simulink model "MultipleAgentsChoice_NoVR"  (R2013b)
settings: Solver=ode45  StartTime=0.0  StopTime=1000  RelTol=1e-4  AbsTol=1e-4
libraries: simulink x24
(part 5 of 5)

== system MultipleAgentsChoice_NoVR/StatePropagation/SatelliteControlAccel/Agent Body3/Actual Thruster response/Ythruster1/Thruster1/ThrustBlock ==
  ForceRequest : Inport
  Short? : Inport  Port=2
  MainSwitch : Inport  Port=3
  Feed : Inport  Port=4
  CathodeEfficiency : Inport  Port=5
  ActiveThruster (logical) : Subsystem
  Bus Creator : BusCreator  Inputs=2
  Product : Product  RndMeth=Zero
  Product1 : Product  RndMeth=Zero
  Voltage/Current : Subsystem
  OutputForce : Outport
  ThrusterData : Outport  Port=2
  wires:
  [CathodeEfficiency] -> Product1/2
  Product/1 -> Product1/1
  [ForceRequest] -> Product/2
  CathodeEfficiency/1 -> [CathodeEfficiency]
  ForceRequest/1 -> [ForceRequest]
  ActiveThruster (logical)/1(Active) -> Product/1
  Bus Creator/1 -> ThrusterData/1
  Voltage/Current/2(Current) -> Bus Creator/2  "current"
  Voltage/Current/1(Voltage) -> Bus Creator/1  "voltage"
  Feed/1 -> ActiveThruster (logical)/3(Feed?), Voltage/Current/3(Feed?)
  Short?/1 -> Voltage/Current/1(Short?), ActiveThruster (logical)/1(Short?)
  MainSwitch/1 -> Voltage/Current/2(MainSwitch), ActiveThruster (logical)/2(ThrusterOn?)
  Product1/1 -> OutputForce/1

== system MultipleAgentsChoice_NoVR/StatePropagation/SatelliteControlAccel/Agent Body3/Actual Thruster response/Zthruster1/Thruster1/ForceShort ==
  note: Detect event and introduce short, otherwise pass through current result of short status
  Event : Inport
  SC : Inport  Port=2
  MainSwitch : Inport  Port=3
  Constant : Constant
  Data Type Conversion : DataTypeConversion
  Detect Increase : simulink/Logic and Bit Operations/Detect Increase  vinit=0  InputProcessing=Inherited  OutDataTypeStr=uint8
  Multiport Switch : MultiPortSwitch  DataPortOrder=Zero-based contiguous  Inputs=2  zeroidx=on
  S/C Conditioning : Subsystem
  SC_out : Outport
  wires:
  Event/1 -> Detect Increase/1
  Detect Increase/1 -> Data Type Conversion/1
  S/C Conditioning/1(Short?) -> SC_out/1
  MainSwitch/1 -> S/C Conditioning/2(MainSwitch)
  Data Type Conversion/1 -> Multiport Switch/1
  SC/1 -> Multiport Switch/2
  Constant/1 -> Multiport Switch/3
  Multiport Switch/1 -> S/C Conditioning/1(SC)

== system MultipleAgentsChoice_NoVR/StatePropagation/SatelliteControlAccel/Agent Body3/Actual Thruster response/Zthruster1/Thruster1/ThrustBlock ==
  ForceRequest : Inport
  Short? : Inport  Port=2
  MainSwitch : Inport  Port=3
  Feed : Inport  Port=4
  CathodeEfficiency : Inport  Port=5
  ActiveThruster (logical) : Subsystem
  Bus Creator : BusCreator  Inputs=2
  Product : Product  RndMeth=Zero
  Product1 : Product  RndMeth=Zero
  Voltage/Current : Subsystem
  OutputForce : Outport
  ThrusterData : Outport  Port=2
  wires:
  MainSwitch/1 -> ActiveThruster (logical)/2(ThrusterOn?), Voltage/Current/2(MainSwitch)
  Short?/1 -> ActiveThruster (logical)/1(Short?), Voltage/Current/1(Short?)
  Feed/1 -> Voltage/Current/3(Feed?), ActiveThruster (logical)/3(Feed?)
  Voltage/Current/1(Voltage) -> Bus Creator/1  "voltage"
  Voltage/Current/2(Current) -> Bus Creator/2  "current"
  Bus Creator/1 -> ThrusterData/1
  ActiveThruster (logical)/1(Active) -> Product/1
  ForceRequest/1 -> [ForceRequest]
  CathodeEfficiency/1 -> [CathodeEfficiency]
  [ForceRequest] -> Product/2
  Product/1 -> Product1/1
  [CathodeEfficiency] -> Product1/2
  Product1/1 -> OutputForce/1

== system MultipleAgentsChoice_NoVR/StatePropagation/SatelliteControlAccel/Agent Body1/Actual Thruster response/XYZthruster/Thruster1/ForceShort/S//C Conditioning ==
  SC : Inport
  MainSwitch : Inport  Port=2
  Constant : Constant  Value=2
  Data Type Conversion : DataTypeConversion
  Detect Decrease : simulink/Logic and Bit Operations/Detect Decrease  vinit=0  InputProcessing=Inherited  OutDataTypeStr=uint8
  Multiport Switch : MultiPortSwitch  DataPortOrder=Zero-based contiguous  Inputs=2  zeroidx=on
  Short? : Outport
  wires:
  MainSwitch/1 -> Detect Decrease/1
  Detect Decrease/1 -> Data Type Conversion/1
  Data Type Conversion/1 -> Multiport Switch/1
  SC/1 -> Multiport Switch/2
  Constant/1 -> Multiport Switch/3
  Multiport Switch/1 -> Short?/1

== system MultipleAgentsChoice_NoVR/StatePropagation/SatelliteControlAccel/Agent Body1/Actual Thruster response/XYZthruster/Thruster1/ThrustBlock/ActiveThruster (logical) ==
  Short? : Inport
  ThrusterOn? : Inport  Port=2
  Feed? : Inport  Port=3
  MATLAB Fcn : MATLABFcn  MATLABFcn=ActiveThruster  OutputDimensions=1
  Mux : Mux  Inputs=3
  Active : Outport
  wires:
  Short?/1 -> Mux/1
  ThrusterOn?/1 -> Mux/2
  Feed?/1 -> Mux/3
  Mux/1 -> MATLAB Fcn/1
  MATLAB Fcn/1 -> Active/1

== system MultipleAgentsChoice_NoVR/StatePropagation/SatelliteControlAccel/Agent Body1/Actual Thruster response/XYZthruster/Thruster1/ThrustBlock/Voltage//Current ==
  Short? : Inport
  MainSwitch : Inport  Port=2
  Feed? : Inport  Port=3
  Demux : Demux  Outputs=2
  MATLAB Fcn : MATLABFcn  MATLABFcn=ThrusterData  OutputDimensions=2
  Mux : Mux  Inputs=3
  Voltage : Outport
  Current : Outport  Port=2
  wires:
  Short?/1 -> Mux/1
  MainSwitch/1 -> Mux/2
  Feed?/1 -> Mux/3
  Mux/1 -> MATLAB Fcn/1
  MATLAB Fcn/1 -> Demux/1
  Demux/1 -> Voltage/1
  Demux/2 -> Current/1

== system MultipleAgentsChoice_NoVR/StatePropagation/SatelliteControlAccel/Agent Body1/Actual Thruster response/Xthruster/Thruster1/ForceShort/S//C Conditioning ==
  SC : Inport
  MainSwitch : Inport  Port=2
  Constant : Constant  Value=2
  Data Type Conversion : DataTypeConversion
  Detect Decrease : simulink/Logic and Bit Operations/Detect Decrease  vinit=0  InputProcessing=Inherited  OutDataTypeStr=uint8
  Multiport Switch : MultiPortSwitch  DataPortOrder=Zero-based contiguous  Inputs=2  zeroidx=on
  Short? : Outport
  wires:
  Multiport Switch/1 -> Short?/1
  Constant/1 -> Multiport Switch/3
  SC/1 -> Multiport Switch/2
  Data Type Conversion/1 -> Multiport Switch/1
  Detect Decrease/1 -> Data Type Conversion/1
  MainSwitch/1 -> Detect Decrease/1

== system MultipleAgentsChoice_NoVR/StatePropagation/SatelliteControlAccel/Agent Body1/Actual Thruster response/Xthruster/Thruster1/ThrustBlock/ActiveThruster (logical) ==
  Short? : Inport
  ThrusterOn? : Inport  Port=2
  Feed? : Inport  Port=3
  MATLAB Fcn : MATLABFcn  MATLABFcn=ActiveThruster  OutputDimensions=1
  Mux : Mux  Inputs=3
  Active : Outport
  wires:
  MATLAB Fcn/1 -> Active/1
  Mux/1 -> MATLAB Fcn/1
  Feed?/1 -> Mux/3
  ThrusterOn?/1 -> Mux/2
  Short?/1 -> Mux/1

== system MultipleAgentsChoice_NoVR/StatePropagation/SatelliteControlAccel/Agent Body1/Actual Thruster response/Xthruster/Thruster1/ThrustBlock/Voltage//Current ==
  Short? : Inport
  MainSwitch : Inport  Port=2
  Feed? : Inport  Port=3
  Demux : Demux  Outputs=2
  MATLAB Fcn : MATLABFcn  MATLABFcn=ThrusterData  OutputDimensions=2
  Mux : Mux  Inputs=3
  Voltage : Outport
  Current : Outport  Port=2
  wires:
  Demux/2 -> Current/1
  Demux/1 -> Voltage/1
  MATLAB Fcn/1 -> Demux/1
  Mux/1 -> MATLAB Fcn/1
  Feed?/1 -> Mux/3
  MainSwitch/1 -> Mux/2
  Short?/1 -> Mux/1

== system MultipleAgentsChoice_NoVR/StatePropagation/SatelliteControlAccel/Agent Body1/Actual Thruster response/Ythruster1/Thruster1/ForceShort/S//C Conditioning ==
  SC : Inport
  MainSwitch : Inport  Port=2
  Constant : Constant  Value=2
  Data Type Conversion : DataTypeConversion
  Detect Decrease : simulink/Logic and Bit Operations/Detect Decrease  vinit=0  InputProcessing=Inherited  OutDataTypeStr=uint8
  Multiport Switch : MultiPortSwitch  DataPortOrder=Zero-based contiguous  Inputs=2  zeroidx=on
  Short? : Outport
  wires:
  MainSwitch/1 -> Detect Decrease/1
  Detect Decrease/1 -> Data Type Conversion/1
  Data Type Conversion/1 -> Multiport Switch/1
  SC/1 -> Multiport Switch/2
  Constant/1 -> Multiport Switch/3
  Multiport Switch/1 -> Short?/1

== system MultipleAgentsChoice_NoVR/StatePropagation/SatelliteControlAccel/Agent Body1/Actual Thruster response/Ythruster1/Thruster1/ThrustBlock/ActiveThruster (logical) ==
  Short? : Inport
  ThrusterOn? : Inport  Port=2
  Feed? : Inport  Port=3
  MATLAB Fcn : MATLABFcn  MATLABFcn=ActiveThruster  OutputDimensions=1
  Mux : Mux  Inputs=3
  Active : Outport
  wires:
  Short?/1 -> Mux/1
  ThrusterOn?/1 -> Mux/2
  Feed?/1 -> Mux/3
  Mux/1 -> MATLAB Fcn/1
  MATLAB Fcn/1 -> Active/1

== system MultipleAgentsChoice_NoVR/StatePropagation/SatelliteControlAccel/Agent Body1/Actual Thruster response/Ythruster1/Thruster1/ThrustBlock/Voltage//Current ==
  Short? : Inport
  MainSwitch : Inport  Port=2
  Feed? : Inport  Port=3
  Demux : Demux  Outputs=2
  MATLAB Fcn : MATLABFcn  MATLABFcn=ThrusterData  OutputDimensions=2
  Mux : Mux  Inputs=3
  Voltage : Outport
  Current : Outport  Port=2
  wires:
  Short?/1 -> Mux/1
  MainSwitch/1 -> Mux/2
  Feed?/1 -> Mux/3
  Mux/1 -> MATLAB Fcn/1
  MATLAB Fcn/1 -> Demux/1
  Demux/1 -> Voltage/1
  Demux/2 -> Current/1

== system MultipleAgentsChoice_NoVR/StatePropagation/SatelliteControlAccel/Agent Body1/Actual Thruster response/Zthruster1/Thruster1/ForceShort/S//C Conditioning ==
  SC : Inport
  MainSwitch : Inport  Port=2
  Constant : Constant  Value=2
  Data Type Conversion : DataTypeConversion
  Detect Decrease : simulink/Logic and Bit Operations/Detect Decrease  vinit=0  InputProcessing=Inherited  OutDataTypeStr=uint8
  Multiport Switch : MultiPortSwitch  DataPortOrder=Zero-based contiguous  Inputs=2  zeroidx=on
  Short? : Outport
  wires:
  Multiport Switch/1 -> Short?/1
  Constant/1 -> Multiport Switch/3
  SC/1 -> Multiport Switch/2
  Data Type Conversion/1 -> Multiport Switch/1
  Detect Decrease/1 -> Data Type Conversion/1
  MainSwitch/1 -> Detect Decrease/1

== system MultipleAgentsChoice_NoVR/StatePropagation/SatelliteControlAccel/Agent Body1/Actual Thruster response/Zthruster1/Thruster1/ThrustBlock/ActiveThruster (logical) ==
  Short? : Inport
  ThrusterOn? : Inport  Port=2
  Feed? : Inport  Port=3
  MATLAB Fcn : MATLABFcn  MATLABFcn=ActiveThruster  OutputDimensions=1
  Mux : Mux  Inputs=3
  Active : Outport
  wires:
  MATLAB Fcn/1 -> Active/1
  Mux/1 -> MATLAB Fcn/1
  Feed?/1 -> Mux/3
  ThrusterOn?/1 -> Mux/2
  Short?/1 -> Mux/1

== system MultipleAgentsChoice_NoVR/StatePropagation/SatelliteControlAccel/Agent Body1/Actual Thruster response/Zthruster1/Thruster1/ThrustBlock/Voltage//Current ==
  Short? : Inport
  MainSwitch : Inport  Port=2
  Feed? : Inport  Port=3
  Demux : Demux  Outputs=2
  MATLAB Fcn : MATLABFcn  MATLABFcn=ThrusterData  OutputDimensions=2
  Mux : Mux  Inputs=3
  Voltage : Outport
  Current : Outport  Port=2
  wires:
  Demux/2 -> Current/1
  Demux/1 -> Voltage/1
  MATLAB Fcn/1 -> Demux/1
  Mux/1 -> MATLAB Fcn/1
  Feed?/1 -> Mux/3
  MainSwitch/1 -> Mux/2
  Short?/1 -> Mux/1

== system MultipleAgentsChoice_NoVR/StatePropagation/SatelliteControlAccel/Agent Body2/Actual Thruster response/XYZthruster/Thruster1/ForceShort/S//C Conditioning ==
  SC : Inport
  MainSwitch : Inport  Port=2
  Constant : Constant  Value=2
  Data Type Conversion : DataTypeConversion
  Detect Decrease : simulink/Logic and Bit Operations/Detect Decrease  vinit=0  InputProcessing=Inherited  OutDataTypeStr=uint8
  Multiport Switch : MultiPortSwitch  DataPortOrder=Zero-based contiguous  Inputs=2  zeroidx=on
  Short? : Outport
  wires:
  Multiport Switch/1 -> Short?/1
  Constant/1 -> Multiport Switch/3
  SC/1 -> Multiport Switch/2
  Data Type Conversion/1 -> Multiport Switch/1
  Detect Decrease/1 -> Data Type Conversion/1
  MainSwitch/1 -> Detect Decrease/1

== system MultipleAgentsChoice_NoVR/StatePropagation/SatelliteControlAccel/Agent Body2/Actual Thruster response/XYZthruster/Thruster1/ThrustBlock/ActiveThruster (logical) ==
  Short? : Inport
  ThrusterOn? : Inport  Port=2
  Feed? : Inport  Port=3
  MATLAB Fcn : MATLABFcn  MATLABFcn=ActiveThruster  OutputDimensions=1
  Mux : Mux  Inputs=3
  Active : Outport
  wires:
  MATLAB Fcn/1 -> Active/1
  Mux/1 -> MATLAB Fcn/1
  Feed?/1 -> Mux/3
  ThrusterOn?/1 -> Mux/2
  Short?/1 -> Mux/1

== system MultipleAgentsChoice_NoVR/StatePropagation/SatelliteControlAccel/Agent Body2/Actual Thruster response/XYZthruster/Thruster1/ThrustBlock/Voltage//Current ==
  Short? : Inport
  MainSwitch : Inport  Port=2
  Feed? : Inport  Port=3
  Demux : Demux  Outputs=2
  MATLAB Fcn : MATLABFcn  MATLABFcn=ThrusterData  OutputDimensions=2
  Mux : Mux  Inputs=3
  Voltage : Outport
  Current : Outport  Port=2
  wires:
  Demux/2 -> Current/1
  Demux/1 -> Voltage/1
  MATLAB Fcn/1 -> Demux/1
  Mux/1 -> MATLAB Fcn/1
  Feed?/1 -> Mux/3
  MainSwitch/1 -> Mux/2
  Short?/1 -> Mux/1

== system MultipleAgentsChoice_NoVR/StatePropagation/SatelliteControlAccel/Agent Body2/Actual Thruster response/Xthruster/Thruster1/ForceShort/S//C Conditioning ==
  SC : Inport
  MainSwitch : Inport  Port=2
  Constant : Constant  Value=2
  Data Type Conversion : DataTypeConversion
  Detect Decrease : simulink/Logic and Bit Operations/Detect Decrease  vinit=0  InputProcessing=Inherited  OutDataTypeStr=uint8
  Multiport Switch : MultiPortSwitch  DataPortOrder=Zero-based contiguous  Inputs=2  zeroidx=on
  Short? : Outport
  wires:
  MainSwitch/1 -> Detect Decrease/1
  Detect Decrease/1 -> Data Type Conversion/1
  Data Type Conversion/1 -> Multiport Switch/1
  SC/1 -> Multiport Switch/2
  Constant/1 -> Multiport Switch/3
  Multiport Switch/1 -> Short?/1

== system MultipleAgentsChoice_NoVR/StatePropagation/SatelliteControlAccel/Agent Body2/Actual Thruster response/Xthruster/Thruster1/ThrustBlock/ActiveThruster (logical) ==
  Short? : Inport
  ThrusterOn? : Inport  Port=2
  Feed? : Inport  Port=3
  MATLAB Fcn : MATLABFcn  MATLABFcn=ActiveThruster  OutputDimensions=1
  Mux : Mux  Inputs=3
  Active : Outport
  wires:
  Short?/1 -> Mux/1
  ThrusterOn?/1 -> Mux/2
  Feed?/1 -> Mux/3
  Mux/1 -> MATLAB Fcn/1
  MATLAB Fcn/1 -> Active/1

== system MultipleAgentsChoice_NoVR/StatePropagation/SatelliteControlAccel/Agent Body2/Actual Thruster response/Xthruster/Thruster1/ThrustBlock/Voltage//Current ==
  Short? : Inport
  MainSwitch : Inport  Port=2
  Feed? : Inport  Port=3
  Demux : Demux  Outputs=2
  MATLAB Fcn : MATLABFcn  MATLABFcn=ThrusterData  OutputDimensions=2
  Mux : Mux  Inputs=3
  Voltage : Outport
  Current : Outport  Port=2
  wires:
  Short?/1 -> Mux/1
  MainSwitch/1 -> Mux/2
  Feed?/1 -> Mux/3
  Mux/1 -> MATLAB Fcn/1
  MATLAB Fcn/1 -> Demux/1
  Demux/1 -> Voltage/1
  Demux/2 -> Current/1

== system MultipleAgentsChoice_NoVR/StatePropagation/SatelliteControlAccel/Agent Body2/Actual Thruster response/Ythruster1/Thruster1/ForceShort/S//C Conditioning ==
  SC : Inport
  MainSwitch : Inport  Port=2
  Constant : Constant  Value=2
  Data Type Conversion : DataTypeConversion
  Detect Decrease : simulink/Logic and Bit Operations/Detect Decrease  vinit=0  InputProcessing=Inherited  OutDataTypeStr=uint8
  Multiport Switch : MultiPortSwitch  DataPortOrder=Zero-based contiguous  Inputs=2  zeroidx=on
  Short? : Outport
  wires:
  Multiport Switch/1 -> Short?/1
  Constant/1 -> Multiport Switch/3
  SC/1 -> Multiport Switch/2
  Data Type Conversion/1 -> Multiport Switch/1
  Detect Decrease/1 -> Data Type Conversion/1
  MainSwitch/1 -> Detect Decrease/1

== system MultipleAgentsChoice_NoVR/StatePropagation/SatelliteControlAccel/Agent Body2/Actual Thruster response/Ythruster1/Thruster1/ThrustBlock/ActiveThruster (logical) ==
  Short? : Inport
  ThrusterOn? : Inport  Port=2
  Feed? : Inport  Port=3
  MATLAB Fcn : MATLABFcn  MATLABFcn=ActiveThruster  OutputDimensions=1
  Mux : Mux  Inputs=3
  Active : Outport
  wires:
  MATLAB Fcn/1 -> Active/1
  Mux/1 -> MATLAB Fcn/1
  Feed?/1 -> Mux/3
  ThrusterOn?/1 -> Mux/2
  Short?/1 -> Mux/1

== system MultipleAgentsChoice_NoVR/StatePropagation/SatelliteControlAccel/Agent Body2/Actual Thruster response/Ythruster1/Thruster1/ThrustBlock/Voltage//Current ==
  Short? : Inport
  MainSwitch : Inport  Port=2
  Feed? : Inport  Port=3
  Demux : Demux  Outputs=2
  MATLAB Fcn : MATLABFcn  MATLABFcn=ThrusterData  OutputDimensions=2
  Mux : Mux  Inputs=3
  Voltage : Outport
  Current : Outport  Port=2
  wires:
  Demux/2 -> Current/1
  Demux/1 -> Voltage/1
  MATLAB Fcn/1 -> Demux/1
  Mux/1 -> MATLAB Fcn/1
  Feed?/1 -> Mux/3
  MainSwitch/1 -> Mux/2
  Short?/1 -> Mux/1

== system MultipleAgentsChoice_NoVR/StatePropagation/SatelliteControlAccel/Agent Body2/Actual Thruster response/Zthruster1/Thruster1/ForceShort/S//C Conditioning ==
  SC : Inport
  MainSwitch : Inport  Port=2
  Constant : Constant  Value=2
  Data Type Conversion : DataTypeConversion
  Detect Decrease : simulink/Logic and Bit Operations/Detect Decrease  vinit=0  InputProcessing=Inherited  OutDataTypeStr=uint8
  Multiport Switch : MultiPortSwitch  DataPortOrder=Zero-based contiguous  Inputs=2  zeroidx=on
  Short? : Outport
  wires:
  MainSwitch/1 -> Detect Decrease/1
  Detect Decrease/1 -> Data Type Conversion/1
  Data Type Conversion/1 -> Multiport Switch/1
  SC/1 -> Multiport Switch/2
  Constant/1 -> Multiport Switch/3
  Multiport Switch/1 -> Short?/1

== system MultipleAgentsChoice_NoVR/StatePropagation/SatelliteControlAccel/Agent Body2/Actual Thruster response/Zthruster1/Thruster1/ThrustBlock/ActiveThruster (logical) ==
  Short? : Inport
  ThrusterOn? : Inport  Port=2
  Feed? : Inport  Port=3
  MATLAB Fcn : MATLABFcn  MATLABFcn=ActiveThruster  OutputDimensions=1
  Mux : Mux  Inputs=3
  Active : Outport
  wires:
  Short?/1 -> Mux/1
  ThrusterOn?/1 -> Mux/2
  Feed?/1 -> Mux/3
  Mux/1 -> MATLAB Fcn/1
  MATLAB Fcn/1 -> Active/1

== system MultipleAgentsChoice_NoVR/StatePropagation/SatelliteControlAccel/Agent Body2/Actual Thruster response/Zthruster1/Thruster1/ThrustBlock/Voltage//Current ==
  Short? : Inport
  MainSwitch : Inport  Port=2
  Feed? : Inport  Port=3
  Demux : Demux  Outputs=2
  MATLAB Fcn : MATLABFcn  MATLABFcn=ThrusterData  OutputDimensions=2
  Mux : Mux  Inputs=3
  Voltage : Outport
  Current : Outport  Port=2
  wires:
  Short?/1 -> Mux/1
  MainSwitch/1 -> Mux/2
  Feed?/1 -> Mux/3
  Mux/1 -> MATLAB Fcn/1
  MATLAB Fcn/1 -> Demux/1
  Demux/1 -> Voltage/1
  Demux/2 -> Current/1

== system MultipleAgentsChoice_NoVR/StatePropagation/SatelliteControlAccel/Agent Body3/Actual Thruster response/XYZthruster/Thruster1/ForceShort/S//C Conditioning ==
  SC : Inport
  MainSwitch : Inport  Port=2
  Constant : Constant  Value=2
  Data Type Conversion : DataTypeConversion
  Detect Decrease : simulink/Logic and Bit Operations/Detect Decrease  vinit=0  InputProcessing=Inherited  OutDataTypeStr=uint8
  Multiport Switch : MultiPortSwitch  DataPortOrder=Zero-based contiguous  Inputs=2  zeroidx=on
  Short? : Outport
  wires:
  Multiport Switch/1 -> Short?/1
  Constant/1 -> Multiport Switch/3
  SC/1 -> Multiport Switch/2
  Data Type Conversion/1 -> Multiport Switch/1
  Detect Decrease/1 -> Data Type Conversion/1
  MainSwitch/1 -> Detect Decrease/1

== system MultipleAgentsChoice_NoVR/StatePropagation/SatelliteControlAccel/Agent Body3/Actual Thruster response/XYZthruster/Thruster1/ThrustBlock/ActiveThruster (logical) ==
  Short? : Inport
  ThrusterOn? : Inport  Port=2
  Feed? : Inport  Port=3
  MATLAB Fcn : MATLABFcn  MATLABFcn=ActiveThruster  OutputDimensions=1
  Mux : Mux  Inputs=3
  Active : Outport
  wires:
  MATLAB Fcn/1 -> Active/1
  Mux/1 -> MATLAB Fcn/1
  Feed?/1 -> Mux/3
  ThrusterOn?/1 -> Mux/2
  Short?/1 -> Mux/1

== system MultipleAgentsChoice_NoVR/StatePropagation/SatelliteControlAccel/Agent Body3/Actual Thruster response/XYZthruster/Thruster1/ThrustBlock/Voltage//Current ==
  Short? : Inport
  MainSwitch : Inport  Port=2
  Feed? : Inport  Port=3
  Demux : Demux  Outputs=2
  MATLAB Fcn : MATLABFcn  MATLABFcn=ThrusterData  OutputDimensions=2
  Mux : Mux  Inputs=3
  Voltage : Outport
  Current : Outport  Port=2
  wires:
  Demux/2 -> Current/1
  Demux/1 -> Voltage/1
  MATLAB Fcn/1 -> Demux/1
  Mux/1 -> MATLAB Fcn/1
  Feed?/1 -> Mux/3
  MainSwitch/1 -> Mux/2
  Short?/1 -> Mux/1

== system MultipleAgentsChoice_NoVR/StatePropagation/SatelliteControlAccel/Agent Body3/Actual Thruster response/Xthruster/Thruster1/ForceShort/S//C Conditioning ==
  SC : Inport
  MainSwitch : Inport  Port=2
  Constant : Constant  Value=2
  Data Type Conversion : DataTypeConversion
  Detect Decrease : simulink/Logic and Bit Operations/Detect Decrease  vinit=0  InputProcessing=Inherited  OutDataTypeStr=uint8
  Multiport Switch : MultiPortSwitch  DataPortOrder=Zero-based contiguous  Inputs=2  zeroidx=on
  Short? : Outport
  wires:
  MainSwitch/1 -> Detect Decrease/1
  Detect Decrease/1 -> Data Type Conversion/1
  Data Type Conversion/1 -> Multiport Switch/1
  SC/1 -> Multiport Switch/2
  Constant/1 -> Multiport Switch/3
  Multiport Switch/1 -> Short?/1

== system MultipleAgentsChoice_NoVR/StatePropagation/SatelliteControlAccel/Agent Body3/Actual Thruster response/Xthruster/Thruster1/ThrustBlock/ActiveThruster (logical) ==
  Short? : Inport
  ThrusterOn? : Inport  Port=2
  Feed? : Inport  Port=3
  MATLAB Fcn : MATLABFcn  MATLABFcn=ActiveThruster  OutputDimensions=1
  Mux : Mux  Inputs=3
  Active : Outport
  wires:
  Short?/1 -> Mux/1
  ThrusterOn?/1 -> Mux/2
  Feed?/1 -> Mux/3
  Mux/1 -> MATLAB Fcn/1
  MATLAB Fcn/1 -> Active/1

== system MultipleAgentsChoice_NoVR/StatePropagation/SatelliteControlAccel/Agent Body3/Actual Thruster response/Xthruster/Thruster1/ThrustBlock/Voltage//Current ==
  Short? : Inport
  MainSwitch : Inport  Port=2
  Feed? : Inport  Port=3
  Demux : Demux  Outputs=2
  MATLAB Fcn : MATLABFcn  MATLABFcn=ThrusterData  OutputDimensions=2
  Mux : Mux  Inputs=3
  Voltage : Outport
  Current : Outport  Port=2
  wires:
  Short?/1 -> Mux/1
  MainSwitch/1 -> Mux/2
  Feed?/1 -> Mux/3
  Mux/1 -> MATLAB Fcn/1
  MATLAB Fcn/1 -> Demux/1
  Demux/1 -> Voltage/1
  Demux/2 -> Current/1

== system MultipleAgentsChoice_NoVR/StatePropagation/SatelliteControlAccel/Agent Body3/Actual Thruster response/Ythruster1/Thruster1/ForceShort/S//C Conditioning ==
  SC : Inport
  MainSwitch : Inport  Port=2
  Constant : Constant  Value=2
  Data Type Conversion : DataTypeConversion
  Detect Decrease : simulink/Logic and Bit Operations/Detect Decrease  vinit=0  InputProcessing=Inherited  OutDataTypeStr=uint8
  Multiport Switch : MultiPortSwitch  DataPortOrder=Zero-based contiguous  Inputs=2  zeroidx=on
  Short? : Outport
  wires:
  Multiport Switch/1 -> Short?/1
  Constant/1 -> Multiport Switch/3
  SC/1 -> Multiport Switch/2
  Data Type Conversion/1 -> Multiport Switch/1
  Detect Decrease/1 -> Data Type Conversion/1
  MainSwitch/1 -> Detect Decrease/1

== system MultipleAgentsChoice_NoVR/StatePropagation/SatelliteControlAccel/Agent Body3/Actual Thruster response/Ythruster1/Thruster1/ThrustBlock/ActiveThruster (logical) ==
  Short? : Inport
  ThrusterOn? : Inport  Port=2
  Feed? : Inport  Port=3
  MATLAB Fcn : MATLABFcn  MATLABFcn=ActiveThruster  OutputDimensions=1
  Mux : Mux  Inputs=3
  Active : Outport
  wires:
  MATLAB Fcn/1 -> Active/1
  Mux/1 -> MATLAB Fcn/1
  Feed?/1 -> Mux/3
  ThrusterOn?/1 -> Mux/2
  Short?/1 -> Mux/1

== system MultipleAgentsChoice_NoVR/StatePropagation/SatelliteControlAccel/Agent Body3/Actual Thruster response/Ythruster1/Thruster1/ThrustBlock/Voltage//Current ==
  Short? : Inport
  MainSwitch : Inport  Port=2
  Feed? : Inport  Port=3
  Demux : Demux  Outputs=2
  MATLAB Fcn : MATLABFcn  MATLABFcn=ThrusterData  OutputDimensions=2
  Mux : Mux  Inputs=3
  Voltage : Outport
  Current : Outport  Port=2
  wires:
  Demux/2 -> Current/1
  Demux/1 -> Voltage/1
  MATLAB Fcn/1 -> Demux/1
  Mux/1 -> MATLAB Fcn/1
  Feed?/1 -> Mux/3
  MainSwitch/1 -> Mux/2
  Short?/1 -> Mux/1

== system MultipleAgentsChoice_NoVR/StatePropagation/SatelliteControlAccel/Agent Body3/Actual Thruster response/Zthruster1/Thruster1/ForceShort/S//C Conditioning ==
  SC : Inport
  MainSwitch : Inport  Port=2
  Constant : Constant  Value=2
  Data Type Conversion : DataTypeConversion
  Detect Decrease : simulink/Logic and Bit Operations/Detect Decrease  vinit=0  InputProcessing=Inherited  OutDataTypeStr=uint8
  Multiport Switch : MultiPortSwitch  DataPortOrder=Zero-based contiguous  Inputs=2  zeroidx=on
  Short? : Outport
  wires:
  MainSwitch/1 -> Detect Decrease/1
  Detect Decrease/1 -> Data Type Conversion/1
  Data Type Conversion/1 -> Multiport Switch/1
  SC/1 -> Multiport Switch/2
  Constant/1 -> Multiport Switch/3
  Multiport Switch/1 -> Short?/1

== system MultipleAgentsChoice_NoVR/StatePropagation/SatelliteControlAccel/Agent Body3/Actual Thruster response/Zthruster1/Thruster1/ThrustBlock/ActiveThruster (logical) ==
  Short? : Inport
  ThrusterOn? : Inport  Port=2
  Feed? : Inport  Port=3
  MATLAB Fcn : MATLABFcn  MATLABFcn=ActiveThruster  OutputDimensions=1
  Mux : Mux  Inputs=3
  Active : Outport
  wires:
  Short?/1 -> Mux/1
  ThrusterOn?/1 -> Mux/2
  Feed?/1 -> Mux/3
  Mux/1 -> MATLAB Fcn/1
  MATLAB Fcn/1 -> Active/1

== system MultipleAgentsChoice_NoVR/StatePropagation/SatelliteControlAccel/Agent Body3/Actual Thruster response/Zthruster1/Thruster1/ThrustBlock/Voltage//Current ==
  Short? : Inport
  MainSwitch : Inport  Port=2
  Feed? : Inport  Port=3
  Demux : Demux  Outputs=2
  MATLAB Fcn : MATLABFcn  MATLABFcn=ThrusterData  OutputDimensions=2
  Mux : Mux  Inputs=3
  Voltage : Outport
  Current : Outport  Port=2
  wires:
  Short?/1 -> Mux/1
  MainSwitch/1 -> Mux/2
  Feed?/1 -> Mux/3
  Mux/1 -> MATLAB Fcn/1
  MATLAB Fcn/1 -> Demux/1
  Demux/1 -> Voltage/1
  Demux/2 -> Current/1
